simulink model "automobilKocenjeBrzinaUdaljenostSimulink"  (R2020a)
settings: Solver=VariableStepAuto  StartTime=0.0  StopTime=10.0  RelTol=1e-3
libraries: simulink x2, fuzblock x1
settings Model: Creator=Hp  LastModifiedBy=Hp

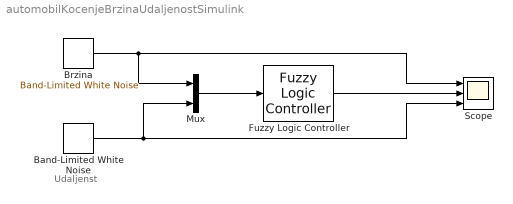
== system automobilKocenjeBrzinaUdaljenostSimulink ==
  note: Udaljenst
  Band-Limited White Noise : simulink/Sources/Band-Limited White Noise  Cov=[150]  Ts=0.1  seed=[23341]
  Brzina : simulink/Sources/Band-Limited White Noise  Cov=[100]  Ts=0.1  seed=[23341]
  Fuzzy Logic Controller : fuzblock/Fuzzy Logic  Controller  FIS=automobilKocenjeBrzinaUdaljenost  OutputSampleNumber=101  DataType=double  FuzzifiedInputs=off  RuleFiringStrengths=off  RuleOutputs=off  AggregatedOutputs=off  SimulateUsing=Interpreted execution  OutOfRangeInputValueMessage=warning  NoRuleFiredMessage=warning  EmptyOutputFuzzySetMessage=warning
  Mux : Mux  Inputs=2
  Scope : Scope  NumInputPorts=3
  wires:
  Mux/1 -> Fuzzy Logic Controller/1
  Brzina/1 -> Scope/1, Mux/1
  Band-Limited White Noise/1 -> Scope/3, Mux/2
  Fuzzy Logic Controller/1 -> Scope/2
